simulink model "dspparameq"  (Simulink 8.3)
settings: Solver=FixedStepDiscrete  SolverMode=SingleTasking  StartTime=0.0  StopTime=inf  RelTol=1e-3
PreLoadFcn:
  | % disp(['Running PreLoadFcn Callback for ' bdroot]);
  | 
  | dspparameq_data
  | 
  | % disp('PreLoadFcn Callback Complete')
StartFcn:
  | % disp(['Running StartFcn Callback for ' bdroot]);
  | 
  | dspparameq_GUI
  | 
  | % disp('StartFcn Callback Complete')
values from neighbouring files (symbols this model uses):
  Fs = AR.SampleRate    [GenDSPTestbenchExample.m]    (also in HelperAircraftKalmanFilter.m = 1000; HelperAudioEqualization.m = 44100; HelperAudioEqualizationCodeGeneration.m = 44100; HelperAudioToneRemoval.m = 44100)
undefined symbols (not defined in the file or in its folder): CoeffsMatrix1, CoeffsMatrix2, CoeffsMatrix3, dfilt, magnitude
libraries: dsparch4 x5, dspsigops x5, dspindex x4, dspxfrm3 x2, dspsrcs4 x1, dspmisc x1, dspsnks4 x1
CloseFcn:
  | % disp(['Running CloseFcn Callback for ' bdroot]);
  | 
  | % Delete parameters
  | clear CoeffsMatrix1 CoeffsMatrix2  CoeffsMatrix3
  | clear coeffsMatrix1   coeffsMatrix2   coeffsMatrix3
  | clear in out
  | 
  | % Delete GUI
  | dspparameq_GUI('close');
  | delete(findall(0, 'type', 'figure', 'Name', 'Three Band Equalizer'));
  | 
  | % disp('CloseFcn Callback Complete')
settings Model: Creator=The MathWorks Inc.
settings SolverCC: PositivePriorityOrder=on
settings DataIOCC: SaveOutput=off  SaveTime=off
settings OptimizationCC: InlineParams=on  InlineInvariantSignals=on  ExpressionDepthLimit=2147483647  ZeroExternalMemoryAtStartup=off  ZeroInternalMemoryAtStartup=off  OptimizeModelRefInitCode=on  LifeSpan=1
settings DebuggingCC: Int32ToFloatConvMsg=none  ParameterPrecisionLossMsg=none  FcnCallInpInsideContextMsg=UseLocalSettings  StrictBusMsg=Warning  LoggingUnavailableSignals=none
settings HardwareCC: ProdLargestAtomicInteger=Long  ProdLargestAtomicFloat=Double  ProdIntDivRoundTo=Zero  ProdEndianess=LittleEndian  ProdHWDeviceType=Analog Devices->Blackfin  TargetHWDeviceType=32-bit Generic
settings SFSimCC: SimParseCustomCode=off
settings RTWCC: SystemTargetFile=ert.tlc  GenCodeOnly=on  GenerateMakefile=off  TemplateMakefile=ert_default_tmf  PostCodeGenCommand=packNGo(buildInfo);  Description=Real-Time Workshop Embedded Coder (no auto configuration)  GenerateReport=on  ProcessScript=ert_make_rtw_hook  IncludeHyperlinkInReport=on  LaunchReport=on  GenerateTraceInfo=on  GenerateTraceReport=on  GenerateTraceReportSl=on  GenerateTraceReportSf=on  GenerateTraceReportEml=on  GenerateCodeInfo=on
settings CodeAppCC: IgnoreCustomStorageClasses=off  SFDataObjDesc=on  CustomSymbolStrType=$N$R$M  CustomCommentsFcn=dspparameq_mpt_comments  InsertBlockDesc=on  EnableCustomComments=on  InternalIdentifier=Classic
settings ERTTargetCC: MultiwordLength=2048  GenerateSampleERTMain=on  IncludeMdlTerminateFcn=off  SuppressErrorStatus=on  SupportAbsoluteTime=off  SupportNonFinite=off  InlinedParameterPlacement=NonHierarchical  ERTSrcFileBannerTemplate=dspparameq_ert_code_template.cgt  ERTCustomFileTemplate=example_file_process.tlc  ConvertIfToSwitch=off  SuppressUnreachableDefaultCases=off

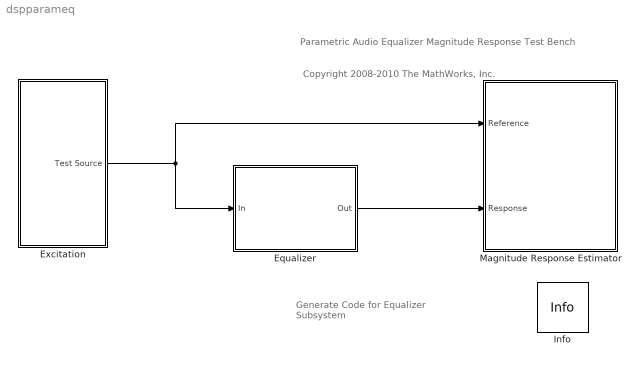
== system dspparameq ==
  note: Generate Code
      | for Equalizer Subsystem
  note: Parametric Audio Equalizer
      | Magnitude Response Test Bench
  note: Copyright 2008-2010 The MathWorks, Inc.
  Equalizer : Subsystem  TreatAsAtomicUnit=on
      mask Display: disp(sprintf('Parametric\nAudio\nEqualizer'))
  Excitation : Subsystem
  Info : dspmisc/Info  SystemSampleTime=-1
  Magnitude Response Estimator : Subsystem
  wires:
  Excitation/1(Test Source) -> Magnitude Response Estimator/1(Reference), Equalizer/1(In)
  Equalizer/1(Out) -> Magnitude Response Estimator/2(Response)

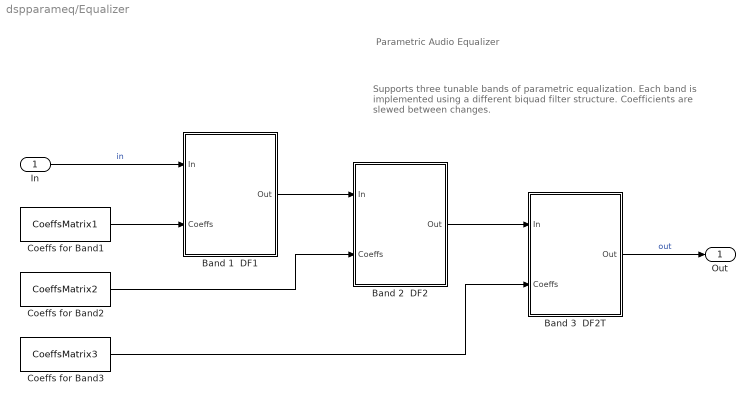
== system dspparameq/Equalizer ==
  note: Parametric Audio Equalizer
  note: Supports three tunable bands of parametric equalization.
      | Each band is implemented using a different biquad filter structure.
      | Coefficients are slewed between changes.
  In : Inport
  Band 1  DF1 : Subsystem  TreatAsAtomicUnit=on
      settings: RTWSystemCode=Nonreusable function
  Band 2  DF2 : Subsystem  TreatAsAtomicUnit=on
      settings: RTWSystemCode=Nonreusable function
  Band 3  DF2T : Subsystem  TreatAsAtomicUnit=on
      settings: RTWSystemCode=Nonreusable function
  Coeffs for Band1 : Constant  Value=CoeffsMatrix1  VectorParams1D=off  OutDataTypeStr=single
  Coeffs for Band2 : Constant  Value=CoeffsMatrix2  VectorParams1D=off  OutDataTypeStr=single
  Coeffs for Band3 : Constant  Value=CoeffsMatrix3  VectorParams1D=off  OutDataTypeStr=single
  Out : Outport
  wires:
  In/1 -> Band 1  DF1/1(In)  "in"
  Coeffs for Band1/1 -> Band 1  DF1/2(Coeffs)
  Band 1  DF1/1(Out) -> Band 2  DF2/1(In)
  Band 2  DF2/1(Out) -> Band 3  DF2T/1(In)
  Band 3  DF2T/1(Out) -> Out/1  "out"
  Coeffs for Band2/1 -> Band 2  DF2/2(Coeffs)
  Coeffs for Band3/1 -> Band 3  DF2T/2(Coeffs)

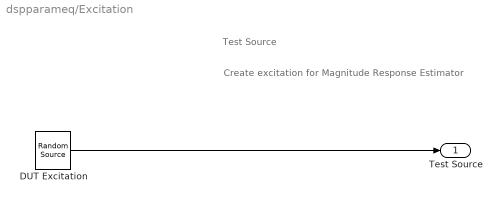
== system dspparameq/Excitation ==
  note: Test Source
  note: Create excitation for Magnitude Response Estimator
  DUT Excitation : dspsrcs4/Random Source  SrcType=Gaussian  NormMethod=Ziggurat  CltLength=12  MinVal=0  MaxVal=1  MeanVal=0  VarVal=1  RepMode=Not repeatable  rawSeed=1  IsInherit=off  SampMode=Discrete  SampTime=1/48000  SampFrame=1024  DataType=Single  OutComplex=Real
  Test Source : Outport
  wires:
  DUT Excitation/1 -> Test Source/1

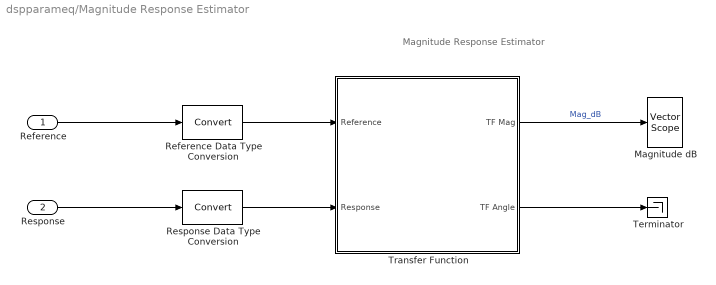
== system dspparameq/Magnitude Response Estimator ==
  note: Magnitude Response Estimator
  Reference : Inport
  Response : Inport  Port=2
  Magnitude dB : dspsnks4/Vector Scope  ScopeProperties=on  Domain=Frequency  HorizSpan=1  DisplayProperties=off  AxisGrid=on  Memory=off  FrameNumber=on  AxisLegend=off  AxisZoom=off  OpenScopeAtSimStart=on  OpenScopeImmediately=off  FigPos=[55 313 372 236]  AxisProperties=off  XUnits=Hertz  XRange=[0...Fs/2]  InheritXIncr=on  XIncr=2*Fs  XLabel=Time  XLimit=User-defined  XMin=0  XMax=22e3  XStart=0  YUnits=dB  YLabel=dB  LineProperties=off  LineColors=[1 0 0]|[0 1 0]  XAxisParamsVer=6.9
      settings: YMin=-16  YMax=16
  Reference Data Type Conversion : DataTypeConversion  SaturateOnIntegerOverflow=on
  Response Data Type Conversion : DataTypeConversion  SaturateOnIntegerOverflow=on
  Terminator : Terminator
  Transfer Function : Subsystem  mask{NFFT=1024, Navg=100, pcnt=100, unwrap_flag=on}
      mask prompts: NFFT "FFT length (power of 2):"; Navg "Spectral Averaging Factor (>=1):"; pcnt "Percentage of  Alias Free Data  (<=100)"; unwrap_flag "Unwrap Phase"
      mask Display: disp('Transfer Function \n Estimation')
  wires:
  Reference/1 -> Reference Data Type Conversion/1
  Response/1 -> Response Data Type Conversion/1
  Transfer Function/1(TF Mag) -> Magnitude dB/1  "Mag_dB"
  Transfer Function/2(TF Angle) -> Terminator/1
  Response Data Type Conversion/1 -> Transfer Function/2(Response)
  Reference Data Type Conversion/1 -> Transfer Function/1(Reference)

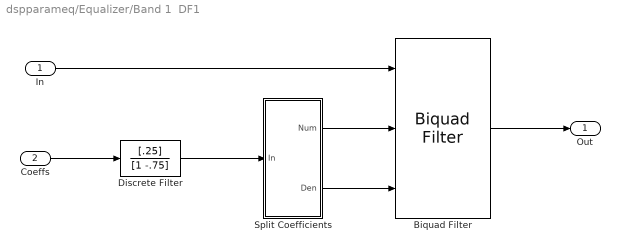
== system dspparameq/Equalizer/Band 1  DF1 ==
  In : Inport
  Coeffs : Inport  Port=2
  Biquad Filter : dsparch4/Biquad Filter  IIRFiltStruct=Direct form I  CoeffSource=Specify via dialog  BiQuadCoeffs=[1 0.3 0.4 1 0.1 0.2]  a0Flag=Warning  IC=0  ICnum=0  ICden=0  InputProcessing=Columns as channels (frame based)  denAccumFracLength=30  denProdOutputFracLength=30  secondMemoryFracLength=15  roundingMode=Floor  overflowMode=off  ScaleValues=1  optimizeScaleValues=on  ScaleValueMode=Assume all are unity and optimize  scaleValueFracLength=14  FilterSource=Input port(s)  dfiltObjectName=dfilt.df2tsos([1 0.3 0.4],[1 0.1 0.2])
      settings: AttributesFormatString=--------------------------------------\n%<IIRFiltStruct>
  Discrete Filter : DiscreteFilter  Numerator=[.25]  Denominator=[1 -.75]
  Split Coefficients : Subsystem
  Out : Outport
  wires:
  Discrete Filter/1 -> Split Coefficients/1(In)
  Biquad Filter/1 -> Out/1
  Coeffs/1 -> Discrete Filter/1
  Split Coefficients/1(Num) -> Biquad Filter/2
  Split Coefficients/2(Den) -> Biquad Filter/3
  In/1 -> Biquad Filter/1

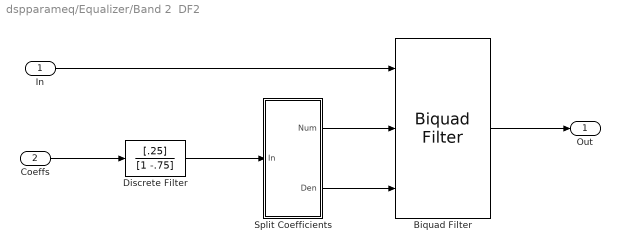
== system dspparameq/Equalizer/Band 2  DF2 ==
  In : Inport
  Coeffs : Inport  Port=2
  Biquad Filter : dsparch4/Biquad Filter  IIRFiltStruct=Direct form II  CoeffSource=Specify via dialog  BiQuadCoeffs=[1 0.3 0.4 1 0.1 0.2]  a0Flag=Warning  IC=0  ICnum=0  ICden=0  InputProcessing=Columns as channels (frame based)  denAccumFracLength=30  denProdOutputFracLength=30  secondMemoryFracLength=15  roundingMode=Floor  overflowMode=off  ScaleValues=1  optimizeScaleValues=on  ScaleValueMode=Assume all are unity and optimize  scaleValueFracLength=14  FilterSource=Input port(s)  dfiltObjectName=dfilt.df2tsos([1 0.3 0.4],[1 0.1 0.2])
      settings: AttributesFormatString=--------------------------------------\n%<IIRFiltStruct>
  Discrete Filter : DiscreteFilter  Numerator=[.25]  Denominator=[1 -.75]
  Split Coefficients : Subsystem
  Out : Outport
  wires:
  Discrete Filter/1 -> Split Coefficients/1(In)
  Biquad Filter/1 -> Out/1
  Coeffs/1 -> Discrete Filter/1
  Split Coefficients/1(Num) -> Biquad Filter/2
  Split Coefficients/2(Den) -> Biquad Filter/3
  In/1 -> Biquad Filter/1

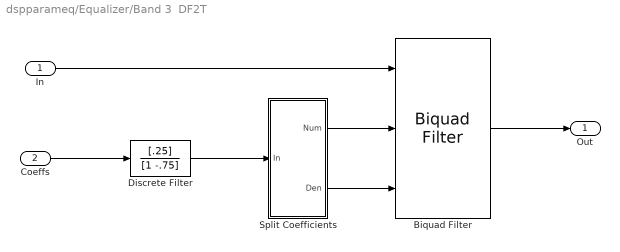
== system dspparameq/Equalizer/Band 3  DF2T ==
  In : Inport
  Coeffs : Inport  Port=2
  Biquad Filter : dsparch4/Biquad Filter  IIRFiltStruct=Direct form II transposed  CoeffSource=Specify via dialog  BiQuadCoeffs=[1 0.3 0.4 1 0.1 0.2]  a0Flag=Warning  IC=0  ICnum=0  ICden=0  InputProcessing=Columns as channels (frame based)  denAccumFracLength=30  denProdOutputFracLength=30  secondMemoryFracLength=15  roundingMode=Floor  overflowMode=off  ScaleValues=1  optimizeScaleValues=on  ScaleValueMode=Assume all are unity and optimize  scaleValueFracLength=14  FilterSource=Input port(s)  dfiltObjectName=dfilt.df2tsos([1 0.3 0.4],[1 0.1 0.2])
      settings: AttributesFormatString=--------------------------------------\n%<IIRFiltStruct>
  Discrete Filter : DiscreteFilter  Numerator=[.25]  Denominator=[1 -.75]
  Split Coefficients : Subsystem
  Out : Outport
  wires:
  Discrete Filter/1 -> Split Coefficients/1(In)
  Biquad Filter/1 -> Out/1
  Coeffs/1 -> Discrete Filter/1
  Split Coefficients/1(Num) -> Biquad Filter/2
  Split Coefficients/2(Den) -> Biquad Filter/3
  In/1 -> Biquad Filter/1

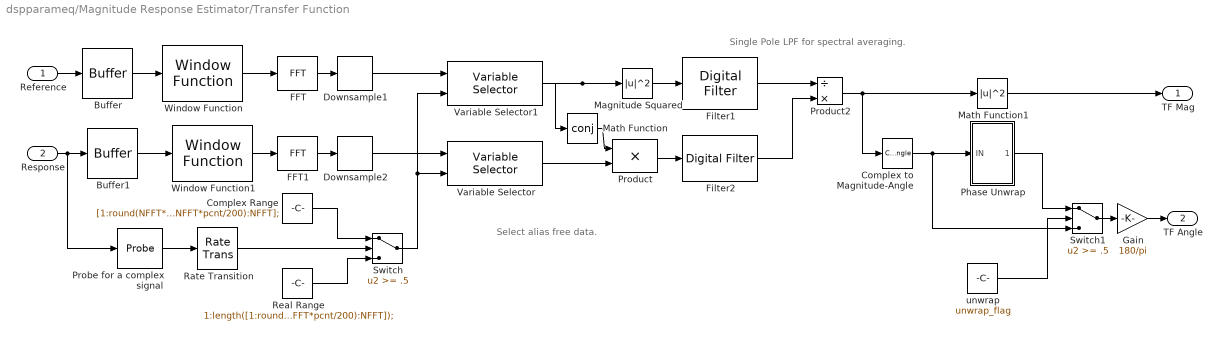
== system dspparameq/Magnitude Response Estimator/Transfer Function ==
  note: Single Pole LPF for spectral averaging.
  note: Select alias free data.
  Reference : Inport
  Response : Inport  Port=2
  Buffer : Buffer  N=NFFT  V=NFFT/2  TreatMby1Signals=One channel
  Buffer1 : Buffer  N=NFFT  V=NFFT/2  TreatMby1Signals=One channel
  Complex Range : Constant  Value=[1:round(NFFT*pcnt/200),round(1+NFFT-NFFT*pcnt/200):NFFT];
  Complex to Magnitude-Angle : ComplexToMagnitudeAngle  Output=Angle
  Downsample1 : dspsigops/Downsample  N=2  phase=0  RateOptions=Allow multirate processing  smode=Allow multirate  fmode=Maintain input frame rate  ic=0
  Downsample2 : dspsigops/Downsample  N=2  phase=0  RateOptions=Allow multirate processing  smode=Allow multirate  fmode=Maintain input frame rate  ic=0
  FFT : dspxfrm3/FFT  CompMethod=Table lookup  TableOpt=NEW  TableOptActive=Speed  BitRevOrder=off  InheritFFTLength=on  FFTLength=64  WrapInput=on  RowConvenienceOn=on  FFTImplementation=Auto  SkipNorm=off  firstCoeffMode=Specify word length  firstCoeffWordLength=16  firstCoeffFracLength=15  firstCoeffDataTypeStr=fixdt(1,16)  firstCoeffLastDataTypeStr=fixdt(1,16)  outputMin=[]  outputMax=[]  roundingMode=Floor  overflowMode=off
  FFT1 : dspxfrm3/FFT  CompMethod=Table lookup  TableOpt=NEW  TableOptActive=Speed  BitRevOrder=off  InheritFFTLength=on  FFTLength=64  WrapInput=on  RowConvenienceOn=on  FFTImplementation=Auto  SkipNorm=off  firstCoeffMode=Specify word length  firstCoeffWordLength=16  firstCoeffFracLength=15  firstCoeffDataTypeStr=fixdt(1,16)  firstCoeffLastDataTypeStr=fixdt(1,16)  outputMin=[]  outputMax=[]  roundingMode=Floor  overflowMode=off
  Filter1 : dsparch4/Digital Filter  TypePopup=IIR (poles & zeros)  IIRFiltStruct=Direct form II transposed  AllPoleFiltStruct=Direct form  FIRFiltStruct=Direct form  CoeffSource=Specify via dialog  NumCoeffs=Navg  DenCoeffs=[Navg -(Navg-1)]/Navg  BiQuadCoeffs=[1 0.3 0.4 1 0.1 0.2]  LatticeCoeffs=[0.2 0.4]  denIgnore=on  FiltPerSampPopup=One filter per frame  IC=eps  ICnum=0  ICden=0  roundingMode=Floor  overflowMode=off  ScaleValues=1  scaleValueFracLength=14  stageInFracLength=15  stageOutFracLength=15  FilterSource=Specify via dialog  dfiltObjectName=dfilt.dffir([1 2 1])
  Filter2 : dsparch4/Digital Filter  TypePopup=IIR (poles & zeros)  IIRFiltStruct=Direct form II transposed  AllPoleFiltStruct=Direct form  FIRFiltStruct=Direct form  CoeffSource=Specify via dialog  NumCoeffs=Navg  DenCoeffs=[Navg -(Navg-1)]/Navg  BiQuadCoeffs=[1 0.3 0.4 1 0.1 0.2]  LatticeCoeffs=[0.2 0.4]  denIgnore=on  FiltPerSampPopup=One filter per frame  IC=eps  ICnum=0  ICden=0  roundingMode=Floor  overflowMode=off  ScaleValues=1  scaleValueFracLength=14  stageInFracLength=15  stageOutFracLength=15  FilterSource=Specify via dialog  dfiltObjectName=dfilt.dffir([1 2 1])
  Gain : Gain  Gain=180/pi
  Magnitude Squared : Math  Operator=magnitude^2  SaturateOnIntegerOverflow=on
  Math Function : Math  Operator=conj  SaturateOnIntegerOverflow=on
  Math Function1 : Math  Operator=magnitude^2  SaturateOnIntegerOverflow=on
  Phase Unwrap : Subsystem
  Probe for a complex signal : Probe  ProbeWidth=off  ProbeSampleTime=off
  Product : Product  SaturateOnIntegerOverflow=on  InputSameDT=on  OutDataTypeStr=Inherit: Same as first input
  Product2 : Product  Inputs=/*  SaturateOnIntegerOverflow=on  InputSameDT=on  OutDataTypeStr=Inherit: Same as first input
  Rate Transition : RateTransition
  Real Range : Constant  Value=1:length([1:round(NFFT*pcnt/200),round(1+NFFT-NFFT*pcnt/200):NFFT]);
  Switch : Switch  Threshold=.5
  Switch1 : Switch  Threshold=.5
  Variable Selector : dspindex/Variable Selector  NumInputs=1  rowsOrCols=Rows  IdxMode=Variable  Elements=[1 3]  ZerOneIdxMode=One-based  errmode=Clip Index  FillMode=on  FillValues=0
  Variable Selector1 : dspindex/Variable Selector  NumInputs=1  rowsOrCols=Rows  IdxMode=Variable  Elements=[1 3]  ZerOneIdxMode=One-based  errmode=Clip Index  FillMode=on  FillValues=0
  Window Function : dspsigops/Window Function  winmode=Apply window to input  wintype=Hann  sampmode=Continuous  samptime=1  N=64  Rs=50  beta=10  winsamp=Periodic  UserWindow=hamming  OptParams=off  UserParams={'symmetric'}  RowConvenienceOn=on  dataType=double  isSigned=on  wordLen=16  udDataType=sfix(16)  fracBitsMode=Best precision  numFracBits=15  roundingMode=Floor  overflowMode=off  numSidelobes=4  sidelobeLevel=-30
  Window Function1 : dspsigops/Window Function  winmode=Apply window to input  wintype=Hann  sampmode=Continuous  samptime=1  N=64  Rs=50  beta=10  winsamp=Periodic  UserWindow=hamming  OptParams=off  UserParams={'symmetric'}  RowConvenienceOn=on  dataType=double  isSigned=on  wordLen=16  udDataType=sfix(16)  fracBitsMode=Best precision  numFracBits=15  roundingMode=Floor  overflowMode=off  numSidelobes=4  sidelobeLevel=-30
  unwrap : Constant  Value=unwrap_flag
  TF Mag : Outport
  TF Angle : Outport  Port=2
  wires:
  Complex Range/1 -> Switch/1
  Real Range/1 -> Switch/3
  Probe for a complex signal/1 -> Rate Transition/1
  Complex to Magnitude-Angle/1 -> Switch1/3, Phase Unwrap/1(IN)
  Gain/1 -> TF Angle/1
  Response/1 -> Buffer1/1, Probe for a complex signal/1
  Reference/1 -> Buffer/1
  Product/1 -> Filter2/1
  FFT1/1 -> Downsample2/1
  Math Function/1 -> Product/1
  Magnitude Squared/1 -> Filter1/1
  FFT/1 -> Downsample1/1
  Math Function1/1 -> TF Mag/1
  Window Function/1 -> FFT/1
  Window Function1/1 -> FFT1/1
  Filter1/1 -> Product2/1
  Filter2/1 -> Product2/2
  Buffer/1 -> Window Function/1
  Buffer1/1 -> Window Function1/1
  Product2/1 -> Math Function1/1, Complex to Magnitude-Angle/1
  Downsample1/1 -> Variable Selector1/1
  Downsample2/1 -> Variable Selector/1
  Variable Selector/1 -> Product/2
  Variable Selector1/1 -> Magnitude Squared/1, Math Function/1
  Rate Transition/1 -> Switch/2
  Switch/1 -> Variable Selector/2, Variable Selector1/2
  Switch1/1 -> Gain/1
  unwrap/1 -> Switch1/2
  Phase Unwrap/1(Out1) -> Switch1/1

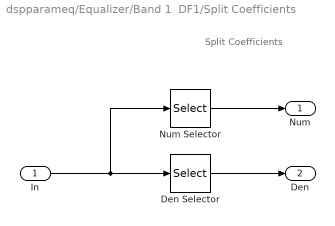
== system dspparameq/Equalizer/Band 1  DF1/Split Coefficients ==
  note: Split Coefficients
  In : Inport
  Den Selector : Selector  InputPortWidth=5  Indices=[4 5]
  Num Selector : Selector  InputPortWidth=5  Indices=[1 2 3]
  Num : Outport
  Den : Outport  Port=2
  wires:
  In/1 -> Num Selector/1, Den Selector/1
  Num Selector/1 -> Num/1
  Den Selector/1 -> Den/1

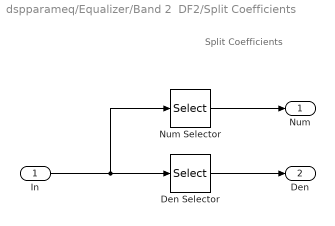
== system dspparameq/Equalizer/Band 2  DF2/Split Coefficients ==
  note: Split Coefficients
  In : Inport
  Den Selector : Selector  InputPortWidth=5  Indices=[4 5]
  Num Selector : Selector  InputPortWidth=5  Indices=[1 2 3]
  Num : Outport
  Den : Outport  Port=2
  wires:
  In/1 -> Num Selector/1, Den Selector/1
  Num Selector/1 -> Num/1
  Den Selector/1 -> Den/1

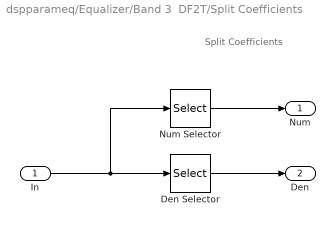
== system dspparameq/Equalizer/Band 3  DF2T/Split Coefficients ==
  note: Split Coefficients
  In : Inport
  Den Selector : Selector  InputPortWidth=5  Indices=[4 5]
  Num Selector : Selector  InputPortWidth=5  Indices=[1 2 3]
  Num : Outport
  Den : Outport  Port=2
  wires:
  In/1 -> Num Selector/1, Den Selector/1
  Num Selector/1 -> Num/1
  Den Selector/1 -> Den/1

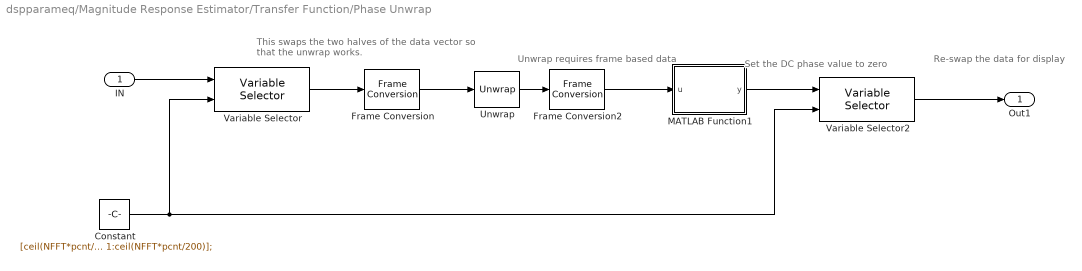
== system dspparameq/Magnitude Response Estimator/Transfer Function/Phase Unwrap ==
  note: This swaps the two halves of the data vector
      | so that the unwrap works.
  note: Set the DC phase value to zero
  note: Re-swap the data for display
  note: Unwrap requires frame based data
  IN : Inport
  Constant : Constant  Value=[ceil(NFFT*pcnt/200)+1:floor(NFFT*pcnt/100) 1:ceil(NFFT*pcnt/200)];
  Frame Conversion : FrameConversion
  Frame Conversion2 : FrameConversion  OutFrame=Sample-based
  MATLAB Function1 : MATLAB Function  TreatAsAtomicUnit=on
  Unwrap : dspsigops/Unwrap  tol=pi  InputProcessing=Columns as channels (frame based)  running=on
  Variable Selector : dspindex/Variable Selector  NumInputs=1  rowsOrCols=Rows  IdxMode=Variable  Elements=[1 3]  ZerOneIdxMode=One-based  errmode=Clip Index  FillMode=on  FillValues=0
  Variable Selector2 : dspindex/Variable Selector  NumInputs=1  rowsOrCols=Rows  IdxMode=Variable  Elements=[1 3]  ZerOneIdxMode=One-based  errmode=Clip Index  FillMode=on  FillValues=0
  Out1 : Outport
  wires:
  Frame Conversion2/1 -> MATLAB Function1/1(u)
  Frame Conversion/1 -> Unwrap/1
  Unwrap/1 -> Frame Conversion2/1
  Variable Selector2/1 -> Out1/1
  IN/1 -> Variable Selector/1
  Constant/1 -> Variable Selector/2, Variable Selector2/2
  Variable Selector/1 -> Frame Conversion/1
  MATLAB Function1/1(y) -> Variable Selector2/1

== matlab function Magnitude Response Estimator/Transfer Function/Phase Unwrap/MATLAB Function1 ==
  data: u input double; y output double
function y = center_sub(u)
% Set Phase to zero at DC.  
y=zeros(size(u));
[r,c]=size(u);
p=ceil(r/2);
for k=1:c
    y(:,k) = u(:,k)-u(p,k);
end;
